simulink model "castor"  (R2021b)
settings: Solver=VariableStepAuto  StartTime=0.0  StopTime=10.0  MaxStep=0.01  RelTol=1e-3
settings Model: Creator=Daniel  LastModifiedBy=Daniel

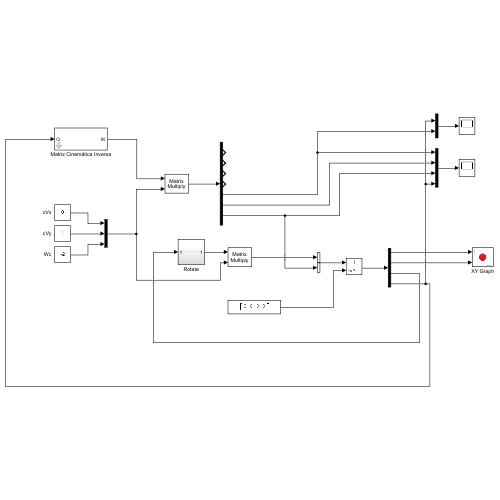
[thumbnail: Simulink's stored preview of the top-level diagram]
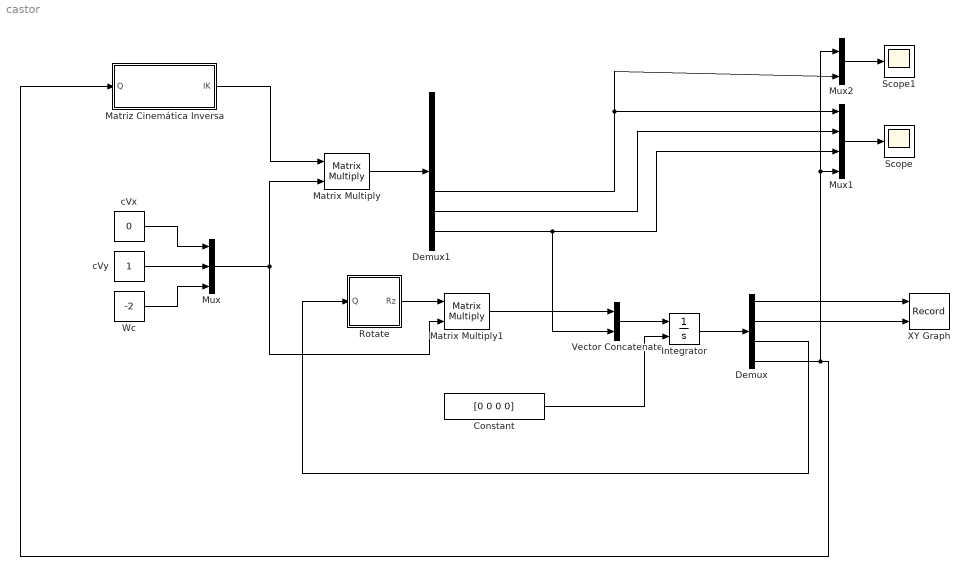
== system castor ==
  Constant : Constant  Value=[0 0 0 0]  VectorParams1D=off  SampleTime=-1
  Demux : Demux
  Demux1 : Demux  Outputs=7
  Integrator : Integrator  InitialConditionSource=external
  Matrix Multiply : Product  Multiplication=Matrix(*)
  Matrix Multiply1 : Product  Multiplication=Matrix(*)
  Matriz Cinemática Inversa : Subsystem  mask{d1=1, d2=1, d3=1}
      mask prompts: d1 "Traction Wheel Offset"; d2 "Steering Offset"; d3 "Steering Length"
  Mux : Mux  Inputs=3
  Mux1 : Mux
  Mux2 : Mux  Inputs=2
  Rotate : Subsystem
  Scope : Scope
  Scope1 : Scope
  Vector Concatenate : Concatenate
  Wc : Constant  Value=-2
  XY Graph : Record  FileSettingsInternal="{\"entries\":[{\"content\":{\"excelSettings\":{\"content\":{},\"type\":\"Streamout.ExcelSettings\"}},\"type\":\"Streamout.FileSettingStorage\",\"uuid\":\"7c3afe2a-d716-4e62-81e4-69494bfe6c2f\"}],\"packageUris\":[\"http://schema.mathworks.com/mf0/streamout_blocks/R2020a\"],\"version\":\"1.0\"}"  Layout=[1 1]  SignalsInternal="{\"entries\":[{\"content\":{\"signals\":[{\"content\":{\"blockPath\":[\"castor/XY Graph\"],\"channel\":[],\"dimensions\":[1,1],\"domain\":\"castor/XY Graph\",\"lineColor\":\"#a2142f\",\"plots\":[1],\"port\":1,\"sid\":[\"\"],\"signalID\":192,\"signalName\":\"Demux:1\"},\"type\":\"RecordBlkView.Signal\",\"uuid\":\"26ce1812-b7d9-4285-be5f-d2145c199b4a\"},{\"content\":{\"blockPath\":[\"castor/XY Graph\"],\"channel\":[],\"dimensions\":[1,1],\"domain\":\"castor/XY Graph\",\"lineColor\":\"#139fff\",\"plots\":[1],\"port\":2,\"sid\":[\"\"],\"signalID\":196,\"signalName\":\"Demux:2\"},\"type\":\"RecordBlkView.Signal\",\"uuid\":\"3dd8047b-72dd-4a14-9d6d-e9049c4f1536\"}]},\"type\":\"RecordBlkView.InputSignals\",\"uuid\":\"a12c8e47-826f-4958-9d42-66ea2b352dbc\"}],\"packageUris\":[\"http://schema.mathworks.com/mf0/streamout_blocks/R2020a\"],\"version\":\"1.0\"}"  VisualizationBindings="{\"xyplotplugin\":{\"info\":[{\"series\":[{\"bindingParametersList\":[{\"parameter\":\"X-Axis\",\"signalID\":192,\"signalName\":\"Demux:1\"},{\"parameter\":\"Y-Axis\",\"signalID\":196,\"signalName\":\"Demux:2\"}],\"seriesID\":23578}],\"subplotID\":1}]}}"  CompatibilityTag=XY
  cVx : Constant  Value=0
  cVy : Constant
  wires:
  cVy/1 -> Mux/2
  cVx/1 -> Mux/1
  Wc/1 -> Mux/3
  Matriz Cinemática Inversa/1(IK) -> Matrix Multiply/1
  Mux/1 -> Matrix Multiply/2, Matrix Multiply1/2
  Vector Concatenate/1 -> Integrator/1
  Integrator/1 -> Demux/1
  Demux/1 -> XY Graph/1
  Demux/2 -> XY Graph/2
  Demux/4 -> Mux2/1, Mux1/4, Matriz Cinemática Inversa/1(Q)
  Matrix Multiply1/1 -> Vector Concatenate/1
  Matrix Multiply/1 -> Demux1/1
  Demux1/7 -> Mux1/3, Vector Concatenate/2
  Demux1/6 -> Mux1/2
  Demux1/5 -> Mux2/2, Mux1/1
  Mux1/1 -> Scope/1
  Mux2/1 -> Scope1/1
  Constant/1 -> Integrator/2
  Rotate/1(Rz) -> Matrix Multiply1/1
  Demux/3 -> Rotate/1(Q)

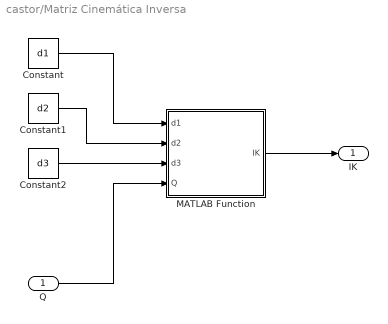
== system castor/Matriz Cinemática Inversa ==
  Q : Inport
  Constant : Constant  Value=d1
  Constant1 : Constant  Value=d2
  Constant2 : Constant  Value=d3
  MATLAB Function : MATLAB Function  TreatAsAtomicUnit=on
  IK : Outport
  wires:
  Constant/1 -> MATLAB Function/1(d1)
  Constant1/1 -> MATLAB Function/2(d2)
  Constant2/1 -> MATLAB Function/3(d3)
  Q/1 -> MATLAB Function/4(Q)
  MATLAB Function/1(IK) -> IK/1

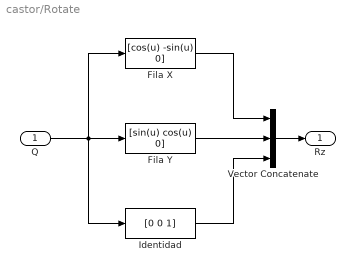
== system castor/Rotate ==
  Q : Inport
  Fila X : MATLABFcn  MATLABFcn=[cos(u) -sin(u) 0]  OutputDimensions=[1 3]  Output1D=off
  Fila Y : MATLABFcn  MATLABFcn=[sin(u) cos(u) 0]  OutputDimensions=[1 3]  Output1D=off
  Identidad : MATLABFcn  MATLABFcn=[0 0 1]  OutputDimensions=[1 3]  Output1D=off
  Vector Concatenate : Concatenate  NumInputs=3  Mode=Multidimensional array
  Rz : Outport
  wires:
  Q/1 -> Identidad/1, Fila Y/1, Fila X/1
  Vector Concatenate/1 -> Rz/1
  Fila Y/1 -> Vector Concatenate/2
  Fila X/1 -> Vector Concatenate/1
  Identidad/1 -> Vector Concatenate/3

== matlab function castor/Matriz Cinemática Inversa/MATLAB Function ==
  data: d1 input; IK output; d2 input; d3 input; Q input
function IK = fcn(d1,d2,d3,Q)

    J1 = [0 0; 1 d1; 0 1];
    J2 = [0 0; 1 -d1; 0 1];
    J3 = [-sin(Q) d2+d3*cos(Q) -d2; cos(Q) d3*sin(Q) 0; 0 1 -1];
    
    % Creación de las matrices A y Jacobiana
    A=[eye(3); eye(3); eye(3)];
    B=[J1 zeros(3,2) zeros(3,3); zeros(3,2) J2 zeros(3,3); zeros(3,2) zeros(3,2) J3];

    IK = inv(B'*B)*B'*A;

end
